simulink subsystem "Encoders"  (R2023b)
settings: Solver=VariableStepAuto  StartTime=0.0  StopTime=10.0  RelTol=1e-3
libraries: simulink x2, arduinosensorlib x2
settings Model: Creator=Enrique  LastModifiedBy=Enrique

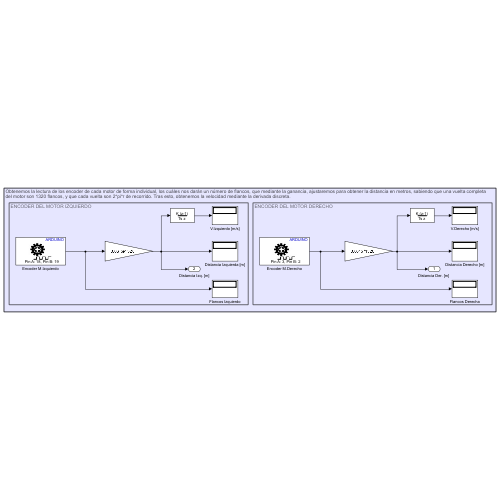
[thumbnail: Simulink's stored preview of the top-level diagram]
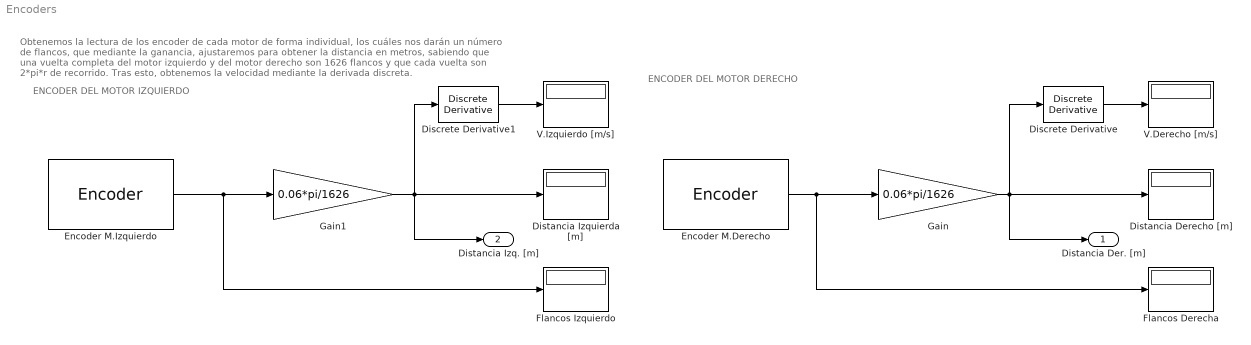
== system Encoders ==
  note: Obtenemos la lectura de los encoder de cada motor de forma individual, los cuáles nos darán un número de flancos, que mediante la ganancia, ajustaremos para obtener la distancia en metros, sabiendo que una vuelta completa
      | del motor izquierdo y del motor derecho son 1626 flancos y que cada vuelta son 2*pi*r de recorrido. Tras esto, obtenemos la velocidad mediante la derivada discreta.
  note: ENCODER DEL MOTOR IZQUIERDO
  note: ENCODER DEL MOTOR DERECHO
  Discrete Derivative : simulink/Discrete/Discrete Derivative  gainval=1.0  ICPrevScaledInput=0.0  OutMin=[]  OutMax=[]  OutDataType=fixdt(1, 16)  OutScaling=2^-10  DoSatur=off
  Discrete Derivative1 : simulink/Discrete/Discrete Derivative  gainval=1.0  ICPrevScaledInput=0.0  OutMin=[]  OutMax=[]  OutDataType=fixdt(1, 16)  OutScaling=2^-10  DoSatur=off
  Distancia Derecho [m] : Display
  Distancia Izquierda [m] : Display
  Encoder M.Derecho : arduinosensorlib/Encoder  InputA=18  InputB=19  Mode=No reset  SampleTime=0.01
  Encoder M.Izquierdo : arduinosensorlib/Encoder  InputA=2  InputB=3  Mode=No reset  SampleTime=0.01
  Flancos Derecha : Display
  Flancos Izquierdo : Display
  Gain : Gain  Gain=0.06*pi/1626  ParamDataTypeStr=double
  Gain1 : Gain  Gain=0.06*pi/1626  ParamDataTypeStr=double
  V.Derecho [m/s] : Display
  V.Izquierdo [m/s] : Display
  "Distancia Der. [m] " : Outport
  Distancia Izq. [m] : Outport  Port=2
  wires:
  Encoder M.Derecho/1 -> Flancos Derecha/1, Gain/1
  Gain/1 -> Distancia Derecho [m]/1, "Distancia Der. [m] "/1, Discrete Derivative/1
  Discrete Derivative/1 -> V.Derecho [m/s]/1
  Discrete Derivative1/1 -> V.Izquierdo [m/s]/1
  Gain1/1 -> Distancia Izq. [m]/1, Discrete Derivative1/1, Distancia Izquierda [m]/1
  Encoder M.Izquierdo/1 -> Flancos Izquierdo/1, Gain1/1
